simulink model "n_trotinettes_crash_discret"  (Simulink 5.1)
settings: Solver=ode45  StartTime=0.0  StopTime=L  RelTol=1e-6
undefined symbols (not defined in the file): Delta, Ig, K, Ka, Ki, Ktach, Kv, L, M_ecart, N, Te
settings Model: LastModifiedBy=acco  BooleanDataType=on  ProdHWDeviceType=Microprocessor

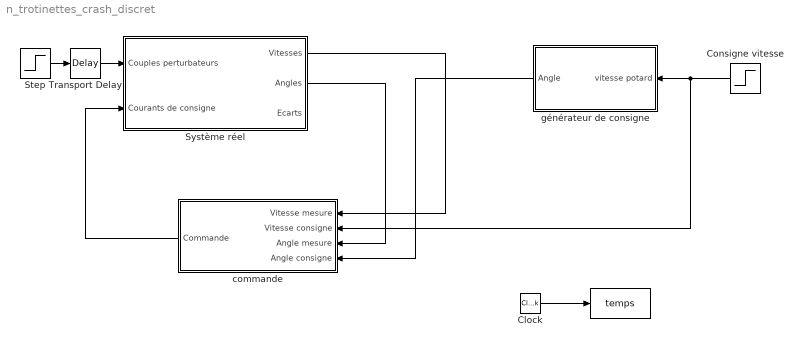
== system n_trotinettes_crash_discret ==
  " " : ToWorkspace  VariableName=temps  SampleTime=-1  SaveFormat=Array
  Clock : DigitalClock  SampleTime=Te
  Consigne vitesse : Step  Orientation=left  Time=L/2  Before=ones(N,1)*0.1  After=ones(N,1)  SampleTime=Te
  Step : Step  Time=L*0.1  Before=zeros(N,1)  After=-ones(N,1)
  Système réel : Subsystem
  Transport Delay : TransportDelay  DelayTime=N-(1:N)
  commande : Subsystem  Orientation=left  TreatAsAtomicUnit=on
      settings: RTWSystemCode=Function  RTWFcnNameOpts=Use subsystem name  RTWFileNameOpts=Use subsystem name
  générateur de consigne : Subsystem  Orientation=left
  wires:
  Step/1 -> Transport Delay/1
  Consigne vitesse/1 -> commande/2(Vitesse consigne), générateur de consigne/1(vitesse potard)
  Système réel/2(Angles) -> commande/3(Angle mesure)
  Clock/1 -> " "/1
  commande/1(Commande) -> Système réel/2(Courants de consigne)
  Système réel/1(Vitesses) -> commande/1(Vitesse mesure)
  générateur de consigne/1(Angle) -> commande/4(Angle consigne)
  Transport Delay/1 -> Système réel/1(Couples perturbateurs)

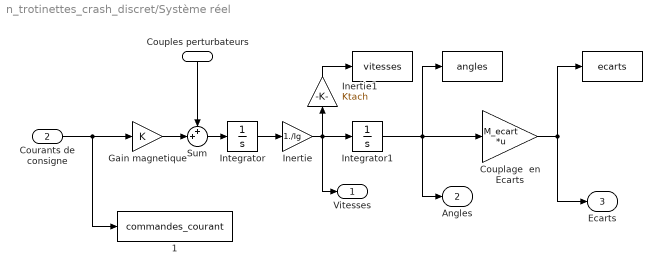
== system n_trotinettes_crash_discret/Système réel ==
  Couples perturbateurs : Inport  Orientation=down  ShowAdditionalParam=on
  Courants de consigne : Inport  Port=2
  " " : ToWorkspace  VariableName=vitesses  SampleTime=Te  SaveFormat=Array
  "  " : ToWorkspace  VariableName=angles  SampleTime=Te  SaveFormat=Array
  "   " : ToWorkspace  VariableName=ecarts  SampleTime=Te  SaveFormat=Array
  "   1" : ToWorkspace  VariableName=commandes_courant  SampleTime=-1  SaveFormat=Array
  Couplage  en Ecarts : Gain  Gain=M_ecart  Multiplication=Matrix(K*u)  SaturateOnIntegerOverflow=on
  Gain magnetique : Gain  Gain=K  SaturateOnIntegerOverflow=on
  Inertie : Gain  Gain=1./Ig  SaturateOnIntegerOverflow=on
  Inertie1 : Gain  Orientation=up  Gain=Ktach  SaturateOnIntegerOverflow=on
  Integrator : Integrator  InitialCondition=zeros(N,1)
  Integrator1 : Integrator  InitialCondition=(0:N-1)*Delta
  Sum : Sum  Inputs=++|  SaturateOnIntegerOverflow=on
  Vitesses : Outport
  Angles : Outport  Port=2
  Ecarts : Outport  Port=3
  wires:
  Integrator/1 -> Inertie/1
  Gain magnetique/1 -> Sum/2
  Sum/1 -> Integrator/1
  Integrator1/1 -> "  "/1, Angles/1, Couplage  en Ecarts/1
  Couples perturbateurs/1 -> Sum/1
  Courants de consigne/1 -> Gain magnetique/1, "   1"/1
  Couplage  en Ecarts/1 -> "   "/1, Ecarts/1
  Inertie/1 -> Vitesses/1, Inertie1/1, Integrator1/1
  Inertie1/1 -> " "/1

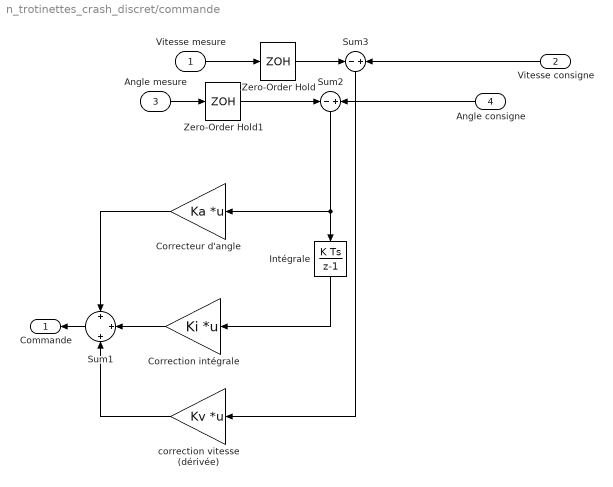
== system n_trotinettes_crash_discret/commande ==
  Vitesse mesure : Inport
  Vitesse consigne : Inport  Orientation=left  Port=2
  Angle mesure : Inport  Port=3
  Angle consigne : Inport  Orientation=left  Port=4
  Correcteur d'angle : Gain  Orientation=left  Gain=Ka  Multiplication=Matrix(K*u)  SaturateOnIntegerOverflow=on
  Correction intégrale : Gain  Orientation=left  Gain=Ki  Multiplication=Matrix(K*u)  SaturateOnIntegerOverflow=on
  Intégrale : DiscreteIntegrator  Orientation=down  InitialCondition=zeros(N,1)  SampleTime=Te
  Sum1 : Sum  Orientation=left  Inputs=+|+|+  SaturateOnIntegerOverflow=on
  Sum2 : Sum  Orientation=down  Inputs=-|+  SaturateOnIntegerOverflow=on
  Sum3 : Sum  Orientation=down  Inputs=-|+  SaturateOnIntegerOverflow=on
  Zero-Order Hold : ZeroOrderHold  SampleTime=Te
  Zero-Order Hold1 : ZeroOrderHold  SampleTime=Te
  correction vitesse (dérivée) : Gain  Orientation=left  Gain=Kv  Multiplication=Matrix(K*u)  SaturateOnIntegerOverflow=on
  Commande : Outport  Orientation=left
  wires:
  Sum2/1 -> Intégrale/1, Correcteur d'angle/1
  Correcteur d'angle/1 -> Sum1/1
  Sum3/1 -> correction vitesse (dérivée)/1
  Intégrale/1 -> Correction intégrale/1
  correction vitesse (dérivée)/1 -> Sum1/3
  Correction intégrale/1 -> Sum1/2
  Vitesse consigne/1 -> Sum3/2
  Angle consigne/1 -> Sum2/2
  Vitesse mesure/1 -> Zero-Order Hold/1
  Angle mesure/1 -> Zero-Order Hold1/1
  Sum1/1 -> Commande/1
  Zero-Order Hold/1 -> Sum3/1
  Zero-Order Hold1/1 -> Sum2/1

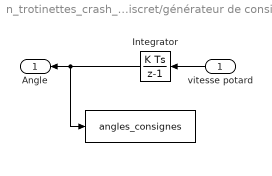
== system n_trotinettes_crash_discret/générateur de consigne ==
  vitesse potard : Inport  Orientation=left
  "  " : ToWorkspace  VariableName=angles_consignes  SampleTime=-1  SaveFormat=Array
  Integrator : DiscreteIntegrator  Orientation=left  InitialCondition=[0:N-1]'*Delta  SampleTime=Te
  Angle : Outport  Orientation=left
  wires:
  Integrator/1 -> "  "/1, Angle/1
  vitesse potard/1 -> Integrator/1
